simulink model "tenzo1_10_lqr0"  (Simulink 7.9)
settings: Solver=ode45  StartTime=0.0  StopTime=10.0  RelTol=1e-3
values from neighbouring files (symbols this model uses):
  AMin = [ ... (first row only)    [AstaTenzo.m]    (also in RiduzioneModello.m = [ 0 1 0 0 0 0 0 0; RiduzioneModello1_05.m = [ 0 1 0 0 0 0 0 0; RiduzioneModello1_10.m = [ 0 1 0 0 0 0 0 0; RiduzioneModello1_15.m)
  Aoss = AMin-V*ClocalMin    [AstaTenzo.m]    (also in RiduzioneModello1_05.m; RiduzioneModello1_10.m; RiduzioneModello1_15.m)
  BMin = [ ... (first row only)    [AstaTenzo.m]    (also in RiduzioneModello.m = [zeros(1,4); RiduzioneModello1_05.m = [zeros(1,4); RiduzioneModello1_10.m = [zeros(1,4); RiduzioneModello1_15.m)
  Boss = [BMin-V*D V M-V*N]    [AstaTenzo.m]    (also in RiduzioneModello1_05.m = [BMin-V*D V]; RiduzioneModello1_10.m = [BMin-V*D V]; RiduzioneModello1_15.m = [BMin-V*D V])
  ClocalMin = [ ... (first row only)    [AstaTenzo.m]    (also in RiduzioneModello.m; RiduzioneModello1_05.m; RiduzioneModello1_10.m; RiduzioneModello1_15.m)
  Coss = eye(n)    [AstaTenzo.m]    (also in RiduzioneModello1_05.m = eye(size(AMin)); RiduzioneModello1_10.m = eye(size(AMin)); RiduzioneModello1_15.m = eye(size(AMin)))
  D = zeros(4,4)    [AstaTenzo.m]    (also in RiduzioneModello.m; RiduzioneModello1_05.m; RiduzioneModello1_10.m; RiduzioneModello1_15.m)
  Doss = zeros(size(Boss))    [AstaTenzo.m]    (also in RiduzioneModello1_05.m; RiduzioneModello1_10.m; RiduzioneModello1_15.m)
  K = lqr(AMin,BMin,Q,R)    [AstaTenzo.m]    (also in RiduzioneModello1_05.m; RiduzioneModello1_10.m; RiduzioneModello1_15.m)
settings Model: Creator=userk  LastModifiedBy=userk

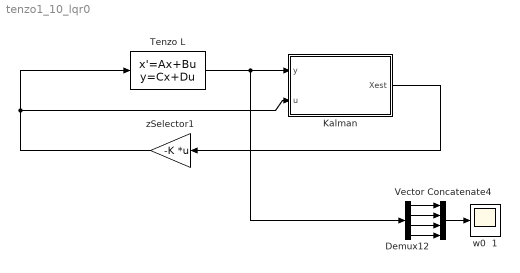
== system tenzo1_10_lqr0 ==
  Demux12 : Demux
  Kalman : Subsystem
  Tenzo L : StateSpace  A=AMin  B=BMin  C=ClocalMin  D=D  X0=[0 0 0 0 0 0 0 0 ]
  Vector Concatenate4 : Concatenate  NumInputs=4
  w0  1 : Scope
      settings: YMin=2500  YMax=7000
  zSelector1 : Gain  Gain=-K  Multiplication=Matrix(K*u)
  wires:
  Demux12/1 -> Vector Concatenate4/1
  Demux12/2 -> Vector Concatenate4/2
  Demux12/3 -> Vector Concatenate4/3
  Demux12/4 -> Vector Concatenate4/4
  Vector Concatenate4/1 -> w0  1/1
  Tenzo L/1 -> Kalman/1(y), Demux12/1
  Kalman/1(Xest) -> zSelector1/1
  zSelector1/1 -> Tenzo L/1, Kalman/2(u)

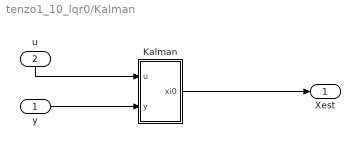
== system tenzo1_10_lqr0/Kalman ==
  y : Inport
  u : Inport  Port=2
  Kalman : Subsystem
  Xest : Outport
  wires:
  y/1 -> Kalman/2(y)
  u/1 -> Kalman/1(u)
  Kalman/1(xi0) -> Xest/1

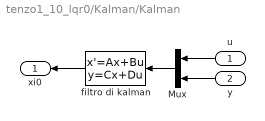
== system tenzo1_10_lqr0/Kalman/Kalman ==
  u : Inport
  y : Inport  Port=2
  Mux : Mux  Inputs=[4 4]
  filtro di kalman : StateSpace  A=Aoss  B=Boss  C=Coss  D=Doss  X0=[0 0 0 0 0 0 0 0]
  xi0 : Outport
  wires:
  y/1 -> Mux/2
  filtro di kalman/1 -> xi0/1
  u/1 -> Mux/1
  Mux/1 -> filtro di kalman/1
